simulink model "evs"  (R2025b)
settings: Solver=ode3  StartTime=0.0  StopTime=10  FixedStep=1e-6  MaxStep=1e-6  RelTol=1e-3
settings Model: SimulationMode=accelerator  Creator=Dell  LastModifiedBy=Dell
settings DataIOCC: SaveOutput=off  SignalLogging=off
settings OptimizationCC: BlockReduction=off  ConditionallyExecuteInputs=off  DefaultParameterBehavior=Inlined
settings DebuggingCC: AlgebraicLoopMsg=error
settings HardwareCC: ProdBitPerPointer=32.0  ProdBitPerSizeT=32.0  ProdBitPerPtrDiffT=32.0  ProdLargestAtomicFloat=None  ProdIntDivRoundTo=Undefined  ProdEndianess=Unspecified  ProdWordSize=32.0  ProdHWDeviceType=ASIC/FPGA->ASIC/FPGA  TargetBitPerPointer=64.0  TargetBitPerSizeT=64.0  TargetBitPerPtrDiffT=64.0  TargetLongLongMode=on  TargetIntDivRoundTo=Zero  TargetEndianess=LittleEndian  TargetWordSize=64.0  TargetHWDeviceType=Custom Processor->MATLAB Host Computer  ProdEqTarget=off

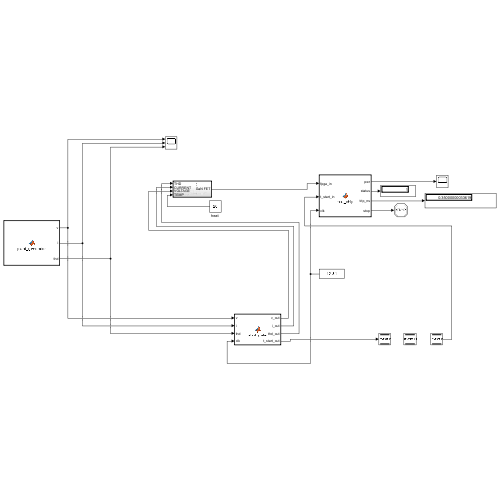
[thumbnail: Simulink's stored preview of the top-level diagram]
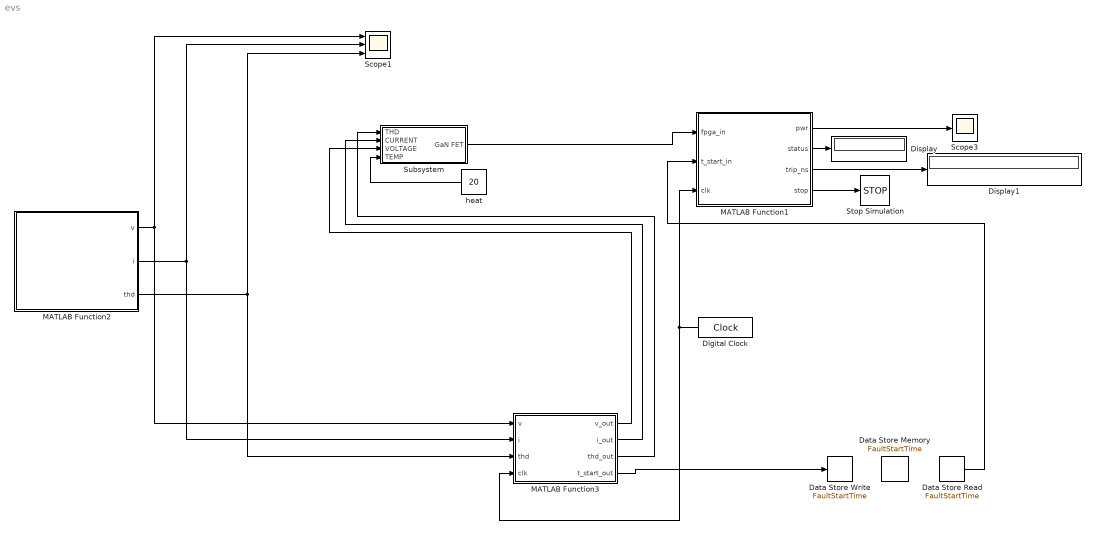
== system evs ==
  Data Store Memory : DataStoreMemory  DataStoreName=FaultStartTime  WriteAfterWriteMsg=warning  ShowAdditionalParam=off
  Data Store Read : DataStoreRead  DataStoreName=FaultStartTime  IndexOptions=Index vector (dialog)  Indices=1  OutputSizes=1
  Data Store Write : DataStoreWrite  DataStoreName=FaultStartTime  IndexOptions=Index vector (dialog)  Indices=1  OutputSizes=1
  Digital Clock : DigitalClock  SampleTime=1e-6
  Display : Display
  Display1 : Display
      settings: Format=decimal (Stored Integer)
  MATLAB Function1 : MATLAB Function  TreatAsAtomicUnit=on
  MATLAB Function2 : MATLAB Function  TreatAsAtomicUnit=on
  MATLAB Function3 : MATLAB Function  TreatAsAtomicUnit=on
  Scope1 : Scope  NumInputPorts=3
      settings: ActiveDisplayYMinimum=-8.200724472385847  ActiveDisplayYMaximum=37.754229060140744
  Scope3 : Scope
      settings: ActiveDisplayYMinimum=0.94772050639605177  ActiveDisplayYMaximum=1.1975611808975719  DataLoggingVariableName=ScopeData3  DataLoggingSaveFormat=Array
  Stop Simulation : Stop
  Subsystem : Subsystem  TreatAsAtomicUnit=on
  "heat " : Constant  Value=20
  wires:
  "heat "/1 -> Subsystem/4(TEMP)
  Subsystem/1(GaN FET) -> MATLAB Function1/1(fpga_in)
  MATLAB Function1/3(trip_ns) -> Display1/1
  MATLAB Function2/1(v) -> Scope1/1, MATLAB Function3/1(v)
  MATLAB Function2/2(i) -> Scope1/2, MATLAB Function3/2(i)
  MATLAB Function2/3(thd) -> Scope1/3, MATLAB Function3/3(thd)
  Digital Clock/1 -> MATLAB Function1/3(clk), MATLAB Function3/4(clk)
  MATLAB Function1/4(stop) -> Stop Simulation/1
  MATLAB Function1/2(status) -> Display/1
  MATLAB Function1/1(pwr) -> Scope3/1
  MATLAB Function3/3(thd_out) -> Subsystem/1(THD)
  MATLAB Function3/2(i_out) -> Subsystem/2(CURRENT)
  MATLAB Function3/1(v_out) -> Subsystem/3(VOLTAGE)
  MATLAB Function3/4(t_start_out) -> Data Store Write/1
  Data Store Read/1 -> MATLAB Function1/2(t_start_in)

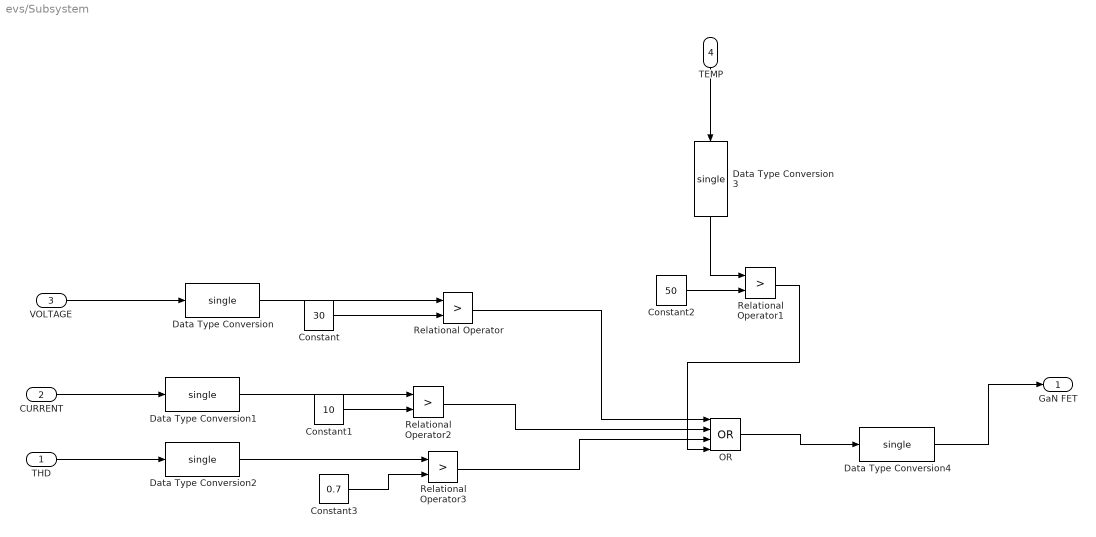
== system evs/Subsystem ==
  THD : Inport
  CURRENT : Inport  Port=2
  VOLTAGE : Inport  Port=3
  TEMP : Inport  Port=4
  Constant : Constant  Value=30
  Constant1 : Constant  Value=10
  Constant2 : Constant  Value=50
  Constant3 : Constant  Value=0.7
  Data Type Conversion{,1..4} (5 alike) : DataTypeConversion  OutDataTypeStr=single  SaturateOnIntegerOverflow=off  RndMeth=Floor
  OR : Logic  Operator=OR  Inputs=4  IconShape=distinctive  AllPortsSameDT=off  OutDataTypeStr=boolean
  Relational Operator{,1..3} (4 alike) : RelationalOperator  Operator=>  OutDataTypeStr=boolean  RndMeth=Simplest  InputSameDT=off
  GaN FET : Outport
  wires:
  VOLTAGE/1 -> Data Type Conversion/1
  TEMP/1 -> Data Type Conversion3/1
  CURRENT/1 -> Data Type Conversion1/1
  THD/1 -> Data Type Conversion2/1
  Data Type Conversion4/1 -> GaN FET/1
  Data Type Conversion/1 -> Relational Operator/1
  Data Type Conversion2/1 -> Relational Operator3/1
  Data Type Conversion1/1 -> Relational Operator2/1
  Data Type Conversion3/1 -> Relational Operator1/1
  Constant/1 -> Relational Operator/2
  Constant1/1 -> Relational Operator2/2
  Constant3/1 -> Relational Operator3/2
  Constant2/1 -> Relational Operator1/2
  Relational Operator/1 -> OR/1
  Relational Operator2/1 -> OR/2
  Relational Operator3/1 -> OR/3
  Relational Operator1/1 -> OR/4
  OR/1 -> Data Type Conversion4/1

== matlab function evs/MATLAB Function1 ==
  data: fpga_in input; t_start_in input; pwr output; status output; trip_ns output; stop output; clk input
function [pwr, status, trip_ns, stop] = mcu_chip(fpga_in, t_start_in, clk)
    persistent trip_latched;
    persistent t_stop_capture;
    persistent stop_counter;
    
    if isempty(trip_latched)
        trip_latched = 0; t_stop_capture = 0; stop_counter = 0;
    end

    % THE SIMPLE CAPTURE: 
    % When FPGA hits 1, we take a snapshot of the current clock
    if fpga_in >= 1 && trip_latched == 0
        t_stop_capture = clk; 
        trip_latched = 1;
    end

    if trip_latched == 1
        % THE CALCULATION: Compare the two snapshots
        % T_Stop (MCU) - T_Start (Sensor) = Total Response Time
        trip_ns = (t_stop_capture - t_start_in) * 1e9;
        
        pwr = 0; 
        status = 1;
        stop_counter = stop_counter + 1;
    else
        % Healthy state: Continuous Square Wave Heartbeat
        pwr = sign(sin(2 * pi * 50 * clk)); 
        status = 0;
        trip_ns = 0;
    end

    stop = (stop_counter > 50);
end

== matlab function evs/MATLAB Function2 ==
  data: v output; i output; thd output
function [v, i, thd] = plant_generator()
    persistent count;
    if isempty(count), count = 1; end
    
    % Thresholds: V=30, I=12, THD=0.75
    N_total = 5000;
    
    % Tight noise level for a stable "DC" look
    % (rand-0.5) keeps the noise centered and small
    v_noise = (rand - 0.5) * 0.4; % Max fluctuation +/- 0.2V
    i_noise = (rand - 0.5) * 0.1; % Max fluctuation +/- 0.05A
    t_noise = (rand - 0.5) * 0.02;% Max fluctuation +/- 0.01
    
    if count == 4920
        % THE ACTUAL HIGH SPIKE (Clearly crossing thresholds)
        v = 40.0; 
        i = 16.0;
        thd = 0.95;
    elseif mod(count, 70) <= 50
        % Stable Medium DC (e.g., 26V is safely below 30V)
        v = 26.0 + v_noise;
        i = 4.0 + i_noise;
        thd = 0.4 + t_noise;
    else
        % Stable Low DC
        v = 22.0 + v_noise;
        i = 1.5 + i_noise;
        thd = 0.1 + t_noise;
    end
    
    if count < N_total
        count = count + 1;
    end
end

== matlab function evs/MATLAB Function3 ==
  data: v input; v_out output; i input; thd input; clk input; i_out output; thd_out output; t_start_out output
function [v_out, i_out, thd_out, t_start_out] = start_gate(v, i, thd, clk)
    persistent t1;
    if isempty(t1), t1 = 0; end

    % Pass-through to Scope
    v_out = v; 
    i_out = i; 
    thd_out = thd;

    % CAPTURE START: Detect fault and apply the 0.35ns buffer
    if (v > 30 || i > 12 || thd > 0.75) && t1 == 0
        % Subtracting 0.35e-9 creates the buffer Jayesh can look for
        t1 = clk - 0.35e-9; 
    end
    
    t_start_out = t1; 
end
